simulink model "simulacion"  (R2021a)
settings: Solver=VariableStepAuto  StartTime=0.0  StopTime=60  RelTol=1e-3
values from neighbouring files (symbols this model uses):
  Gf = tf(FuncionDeTransferencia.numerator,FuncionDeTransferencia.denominator)    [desarrollo.m]
  Gt = tf(FuncionDeTransferencia.numerator,FuncionDeTransferencia.denominator)    [desarrollo.m]
  Kd1 = K    [desarrollo.m]
  Ki2 = Gc2.num{1}(2)    [desarrollo.m]
  Kp1 = K*zero    [desarrollo.m]
  Kp2 = Gc2.num{1}(1)    [desarrollo.m]
settings Model: Creator=pierr  LastModifiedBy=pierr

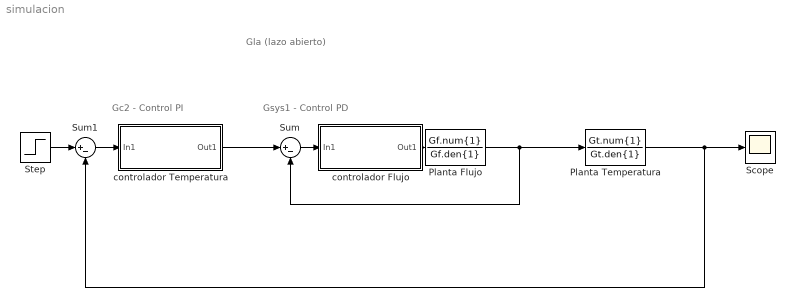
== system simulacion ==
  note: Gc2 - Control PI
  note: Gla (lazo abierto)
  note: Gsys1 - Control PD
  Planta Flujo : TransferFcn  Numerator=Gf.num{1}  Denominator=Gf.den{1}
  Planta Temperatura : TransferFcn  Numerator=Gt.num{1}  Denominator=Gt.den{1}
  Scope : Scope
  Step : Step  Time=0  After=27  SampleTime=0
  Sum : Sum  Inputs=|+-
  Sum1 : Sum  Inputs=|+-
  controlador Flujo : Subsystem
  controlador Temperatura : Subsystem
  wires:
  controlador Flujo/1(Out1) -> Planta Flujo/1
  Sum/1 -> controlador Flujo/1(In1)
  controlador Temperatura/1(Out1) -> Sum/1
  Sum1/1 -> controlador Temperatura/1(In1)
  Step/1 -> Sum1/1
  Planta Flujo/1 -> Sum/2, Planta Temperatura/1
  Planta Temperatura/1 -> Sum1/2, Scope/1

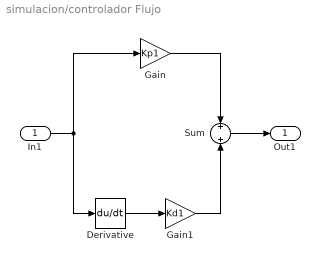
== system simulacion/controlador Flujo ==
  In1 : Inport
  Derivative : Derivative
  Gain : Gain  Gain=Kp1
  Gain1 : Gain  Gain=Kd1
  Sum : Sum  Inputs=+||+
  Out1 : Outport
  wires:
  Sum/1 -> Out1/1
  Derivative/1 -> Gain1/1
  In1/1 -> Derivative/1, Gain/1
  Gain/1 -> Sum/1
  Gain1/1 -> Sum/2

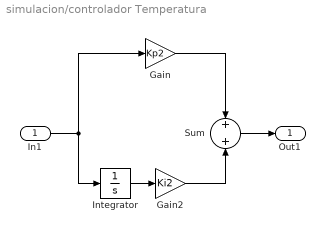
== system simulacion/controlador Temperatura ==
  In1 : Inport
  Gain : Gain  Gain=Kp2
  Gain2 : Gain  Gain=Ki2
  Integrator : Integrator
  Sum : Sum  Inputs=+|+
  Out1 : Outport
  wires:
  Sum/1 -> Out1/1
  Gain/1 -> Sum/1
  In1/1 -> Integrator/1, Gain/1
  Integrator/1 -> Gain2/1
  Gain2/1 -> Sum/2
